simulink model "Parent_Model"  (R2014a)
settings: Solver=FixedStepDiscrete  StartTime=0.0  StopTime=10.0  FixedStep=1/400  RelTol=1e-3
settings Model: Creator=darenlee  LastModifiedBy=darenlee
settings SolverCC: PositivePriorityOrder=on
settings OptimizationCC: OptimizeModelRefInitCode=on  LifeSpan=1  MaxStackSize=64
settings HardwareCC: ProdLargestAtomicInteger=Long  ProdLargestAtomicFloat=Double  ProdEndianess=LittleEndian  ProdHWDeviceType=ARM Compatible->ARM Cortex
settings RTWCC: SystemTargetFile=ert.tlc  TLCOptions=-aInlineSetEventsForThisBaseRateFcn=TLC_FALSE -aSuppressMultiTaskScheduler=TLC_FALSE  TemplateMakefile=ert_default_tmf  Description=Embedded Coder  GenerateReport=on  ProcessScript=ert_make_rtw_hook  Toolchain=Code Sourcery  IncludeHyperlinkInReport=on  LaunchReport=on  CodeExecutionProfiling=on  CodeProfilingSaveOptions=AllData  CodeProfilingInstrumentation=on  GenerateTraceInfo=on  GenerateTraceReport=on  GenerateTraceReportSl=on  GenerateTraceReportSf=on  GenerateTraceReportEml=on  GenerateCodeReplacementReport=on
settings CodeAppCC: IgnoreCustomStorageClasses=off
settings ERTTargetCC: CodeReplacementLibrary=GCC ARM Cortex-A9  ParMdlRefBuildCompliant=on  CompOptLevelCompliant=on  ConcurrentExecutionCompliant=on  ERTFirstTimeCompliant=on  ModelStepFunctionPrototypeControlCompliant=on  CPPClassGenCompliant=on  InlinedParameterPlacement=Hierarchical

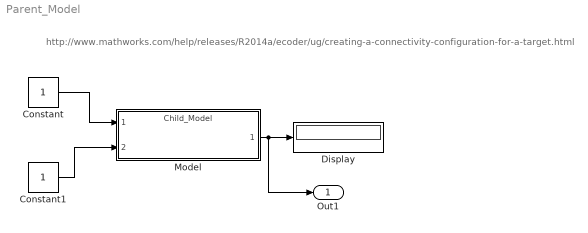
== system Parent_Model ==
  note: http://www.mathworks.com/help/releases/R2014a/ecoder/ug/creating-a-connectivity-configuration-for-a-target.html
  Constant : Constant
  Constant1 : Constant
  Display : Display
  Model : ModelReference  ModelNameDialog=Child_Model.slx  SimulationMode=Processor-in-the-loop (PIL)  ModelReferenceVersion=1.16  CopyOfModelName=Child_Model.slx  DefaultDataLogging=on
  Out1 : Outport
  wires:
  Constant/1 -> Model/1
  Constant1/1 -> Model/2
  Model/1 -> Out1/1, Display/1
